simulink model "r2_deng_tvg"  (R2012b)
(part 3 of 46)

      mask prompts: io_dir "I/O direction"; io_delay "I/O delay"; sample_period "Sample period"; names "Name:"; bitwidths "Bitwidth:"; arith_types "Type (ufix=0, fix=1, bool=2):"; bin_pts "Binary pt:"; show_format "Print format string?"
      mask init:
      | swreg_init(gcb)
      settings: AttributesFormatString=1input:uf32.0,
      mask TypeOptions mode: one value | fields of equal size | fields of arbitrary size
      mask Callback mode: swreg_cb(gcb);
      mask TypeOptions io_dir: To Processor | From Processor
      mask Callback io_dir:
      | mask_enables = get_param(gcb, 'MaskEnables');
      | mask_names = get_param(gcb, 'MaskNames');
      | if strcmp(get_param(gcb, 'io_dir'), 'To Processor'),
      |     mask_enables{ismember(mask_names, 'sample_period')} = 'off';
      | else
      |     mask_enables{ismember(mask_names, 'sample_period')} = 'on';
      | end
      | set_param(gcb, 'MaskEnables', mask_enables);
      mask Callback bitwidths:
      | blk = gcb;
      | mode = get_param(blk, 'mode');
      | current_widths = eval(get_param(blk, 'bitwidths'));
      | if (strcmp(mode, 'one value') || strcmp(mode, 'fields of equal size')) && (length(current_widths) > 1),
      |     error('Only one width may be specified for this mode.');
      | elseif strcmp(mode, 'fields of arbitrary size')
      |     current_names = textscan(strtrim(strrep(strrep(get_param(blk, 'names'), ']', ''), '[', '')), '%s');
      |     current_names = current_names{1};
      |     numios = length(current_names);
      |     if length(current_widths) ~= numios,
      |         error('%d field names specified, but %d widths?', numios, length(current_widths));
      |     end
      | end
      | total_width = 0;
      | for ctr = 1 : length(current_widths),
      |     total_width = total_width + current_widths(ctr);
      | end
      | if total_width > 32,
      |     error('Total width must be 32 or less, set to %d.', total_width);
      | end
      mask Callback arith_types:
      | blk = gcb;
      | mode = get_param(blk, 'mode');
      | current_types = eval(get_param(blk, 'arith_types'));
      | numios = length(current_types);
      | if (strcmp(mode, 'one value') || strcmp(mode, 'fields of equal size')) && (length(current_types) > 1),
      |     error('Only one type may be specified for this mode.');
      | elseif strcmp(mode, 'fields of arbitrary size')
      |     current_names = textscan(strtrim(strrep(strrep(get_param(blk, 'names'), ']', ''), '[', '')), '%s');
      |     current_names = current_names{1};
      |     numios = length(current_names);
      |     if length(current_types) ~= numios,
      |         error('%d field names specified, but %d types?', numios, length(current_types));
      |     end
      | end
      | problem = 0;
      | for ctr = 1 : numios,
      |     t = current_types(ctr);
      |     if (t < 0) || (t > 2),
      |         problem = t;
      |         ctr = numios + 1;
      |     end
      | end
      | if problem ~= 0,
      |     error('Type cannot be %i, must be 0, 1 or 2.', problem);
      | end
      mask Callback bin_pts:
      | blk = gcb;
      | mode = get_param(blk, 'mode');
      | current_bins = eval(get_param(blk, 'bin_pts'));
      | if (strcmp(mode, 'one value') || strcmp(mode, 'fields of equal size')) && (length(current_bins) > 1),
      |     error('Only one binary pt may be specified for this mode.');
      | elseif strcmp(mode, 'fields of arbitrary size')
      |     current_names = textscan(strtrim(strrep(strrep(get_param(blk, 'names'), ']', ''), '[', '')), '%s');
      |     current_names = current_names{1};
      |     numios = length(current_names);
      |     if length(current_bins) ~= numios,
      |         error('%d field names specified, but %d binary pts?', numios, length(current_bins));
      |     end
      | end
  tick_offset_msw : Subsystem  Tag=xps:sw_reg  AncestorBlock=xps_library/software register  mask(swreg){mode=one value, io_dir=From Processor, io_delay=1, sample_period=1, names=reg, bitwidths=32, arith_types=0, bin_pts=0, show_format=on}
      mask prompts: io_dir "I/O direction"; io_delay "I/O delay"; sample_period "Sample period"; names "Name:"; bitwidths "Bitwidth:"; arith_types "Type (ufix=0, fix=1, bool=2):"; bin_pts "Binary pt:"; show_format "Print format string?"
      mask init:
      | swreg_init(gcb)
      settings: AttributesFormatString=1input:uf32.0,
      mask TypeOptions mode: one value | fields of equal size | fields of arbitrary size
      mask Callback mode: swreg_cb(gcb);
      mask TypeOptions io_dir: To Processor | From Processor
      mask Callback io_dir:
      | mask_enables = get_param(gcb, 'MaskEnables');
      | mask_names = get_param(gcb, 'MaskNames');
      | if strcmp(get_param(gcb, 'io_dir'), 'To Processor'),
      |     mask_enables{ismember(mask_names, 'sample_period')} = 'off';
      | else
      |     mask_enables{ismember(mask_names, 'sample_period')} = 'on';
      | end
      | set_param(gcb, 'MaskEnables', mask_enables);
      mask Callback bitwidths:
      | blk = gcb;
      | mode = get_param(blk, 'mode');
      | current_widths = eval(get_param(blk, 'bitwidths'));
      | if (strcmp(mode, 'one value') || strcmp(mode, 'fields of equal size')) && (length(current_widths) > 1),
      |     error('Only one width may be specified for this mode.');
      | elseif strcmp(mode, 'fields of arbitrary size')
      |     current_names = textscan(strtrim(strrep(strrep(get_param(blk, 'names'), ']', ''), '[', '')), '%s');
      |     current_names = current_names{1};
      |     numios = length(current_names);
      |     if length(current_widths) ~= numios,
      |         error('%d field names specified, but %d widths?', numios, length(current_widths));
      |     end
      | end
      | total_width = 0;
      | for ctr = 1 : length(current_widths),
      |     total_width = total_width + current_widths(ctr);
      | end
      | if total_width > 32,
      |     error('Total width must be 32 or less, set to %d.', total_width);
      | end
      mask Callback arith_types:
      | blk = gcb;
      | mode = get_param(blk, 'mode');
      | current_types = eval(get_param(blk, 'arith_types'));
      | numios = length(current_types);
      | if (strcmp(mode, 'one value') || strcmp(mode, 'fields of equal size')) && (length(current_types) > 1),
      |     error('Only one type may be specified for this mode.');
      | elseif strcmp(mode, 'fields of arbitrary size')
      |     current_names = textscan(strtrim(strrep(strrep(get_param(blk, 'names'), ']', ''), '[', '')), '%s');
      |     current_names = current_names{1};
      |     numios = length(current_names);
      |     if length(current_types) ~= numios,
      |         error('%d field names specified, but %d types?', numios, length(current_types));
      |     end
      | end
      | problem = 0;
      | for ctr = 1 : numios,
      |     t = current_types(ctr);
      |     if (t < 0) || (t > 2),
      |         problem = t;
      |         ctr = numios + 1;
      |     end
      | end
      | if problem ~= 0,
      |     error('Type cannot be %i, must be 0, 1 or 2.', problem);
      | end
      mask Callback bin_pts:
      | blk = gcb;
      | mode = get_param(blk, 'mode');
      | current_bins = eval(get_param(blk, 'bin_pts'));
      | if (strcmp(mode, 'one value') || strcmp(mode, 'fields of equal size')) && (length(current_bins) > 1),
      |     error('Only one binary pt may be specified for this mode.');
      | elseif strcmp(mode, 'fields of arbitrary size')
      |     current_names = textscan(strtrim(strrep(strrep(get_param(blk, 'names'), ']', ''), '[', '')), '%s');
      |     current_names = current_names{1};
      |     numios = length(current_names);
      |     if length(current_bins) ~= numios,
      |         error('%d field names specified, but %d binary pts?', numios, length(current_bins));
      |     end
      | end
  ticks_since_mrst : Subsystem
  tvg_spead_time_with_pkt_ctr : Subsystem  mask{packetlen_bits=9}
      mask prompts: packetlen_bits "Packet length, num 80-bit words (2^?):"
  wng0 : Subsystem
  wng1 : Subsystem
  wng_corr : Subsystem
  xsg : xps_library/XSG core config  Tag=xps:xsg  hw_sys=ROACH2:sx475t  clk_src=sys_clk  ROACH_clk_src=sys_clk  ROACH2_clk_src=sys_clk  MKDIG_clk_src=sys_clk  clk_rate=1712/8  sample_period=1  synthesis_tool=XST
  tag scope: local_time=global, spead_data0=global, spead_data1=global, spead_data2=global, spead_data3=global, spead_eof0=global, spead_eof1=global, spead_eof2=global, spead_eof3=global, spead_valid0=global, spead_valid1=global, spead_valid2=global, spead_valid3=global, up_cnt_rst=global
  wires:
  [tvg_select0] -> Delay102/1
  Mux/1 -> Assert/1  "d80_0"
  fifo0/1(fifo_data80) -> pipeline96/1(d)  "data00"
  fifo0/2(fifo_dv) -> Gateway Out/1, pipeline97/1(d)  "dv00"
  fifo0/3(word_start) -> Gateway Out2/1, pipeline98/1(d)  "ws00"
  fifo0/4(pkt_start) -> Gateway Out4/1, pipeline99/1(d)  "ps00"
  gbe_porttx/1(in_reg) -> pipeline16/1(d), pipeline15/1(d)
  Constant9/1 -> gbe_porttx/1(sim_1)
  Constant10/1 -> gbe_iptx0/1(sim_1)
  Constant12/1 -> gbe_iptx1/1(sim_1)
  Constant13/1 -> gbe_iptx2/1(sim_1)
  Constant14/1 -> gbe_iptx3/1(sim_1)
  Constant15/1 -> digitiser_id/1(sim_1)
  Constant17/1 -> receptor_id/1(sim_1)
  fifo0/5(fifo_full) -> Terminator16/1  "full00"
  fifo0/6(fifo_empty) -> Terminator23/1  "empty00"
  fifo1/1(fifo_data80) -> pipeline100/1(d)  "data01"
  fifo1/2(fifo_dv) -> Gateway Out1/1, pipeline101/1(d)  "dv01"
  fifo1/3(word_start) -> Gateway Out3/1, pipeline102/1(d)  "ws01"
  fifo1/4(pkt_start) -> Gateway Out5/1, pipeline103/1(d)  "ps01"
  pack_80_64_01/3(data64) -> pipeline117/1(d)  "d64_00"
  pack_80_64_01/2(valid64) -> pipeline116/1(d)  "v64_01"
  pack_80_64_01/1(ready64) -> pipeline115/1(d)  "r64_01"
  fifo1/5(fifo_full) -> Terminator18/1
  fifo1/6(fifo_empty) -> Terminator20/1
  Inverter/1 -> fifo1/2(fifo_we_en)
  Constant16/1 -> digitiser_id/2(sim_2)
  receptor_id/1(in_receptor_id) -> bus_create/3(in3)
  Constant6/1 -> receptor_id/2(sim_2)
  Constant19/1 -> receptor_id/3(sim_3)
  [hdr_0x3101] -> bus_create9/1(in1)
  [pol0_id] -> bus_create9/2(in2)
  [hdr_0x3101] -> bus_create1/1(in1)
  [pol0_id] -> bus_create1/2(in2)
  [speadtime0] -> spead_pack0/8(hdr5_0x1600_DIR), spead_pack0/4(hdr_heap_id)  "timein0"
  bus_create9/1(bus_out) -> spead_pack0/9(hdr6_0x3101_DIR)
  [status0] -> spead_pack0/10(hdr7_0x3102_DIR)
  bus_create1/1(bus_out) -> spead_pack1/9(hdr6_0x3101_DIR)
  [status1] -> spead_pack1/10(hdr7_0x3102_DIR)
  Mux3/1 -> Delay10/1, Delay11/1, Delay12/1, Delay1/1  "status0"
  [tvg_ltime] -> fifo_select/1(localtime)
  fifo_select/1(select) -> Delay3/1  "fifo_select"
  Delay3/1 -> [fifoselect], Inverter/1, fifo0/2(fifo_we_en)  "fifoselect"
  [speadtime1] -> spead_pack1/4(hdr_heap_id), spead_pack1/8(hdr5_0x1600_DIR)  "timein1"
  pack_80_64_00/1(ready64) -> pipeline112/1(d)  "r64_00"
  pack_80_64_00/2(valid64) -> pipeline113/1(d)  "v64_00"
  pack_80_64_00/3(data64) -> pipeline114/1(d)  "d64_00"
  [spead_heapsize] -> spead_pack0/5(hdr_heap_size)
  [spead_heapoffset] -> spead_pack0/6(hdr_heap_offset)
  [spead_pktlen] -> spead_pack0/7(hdr_pkt_len_words)
  [spead_heapsize] -> spead_pack1/5(hdr_heap_size)
  [spead_heapoffset] -> spead_pack1/6(hdr_heap_offset)
  [spead_pktlen] -> spead_pack1/7(hdr_pkt_len_words)
  [masked_time] -> Delay128/1
  Assert/1 -> fifo1/1(data80), fifo0/1(data80)
  tvg_spead_time_with_pkt_ctr/1(local_time) -> Delay131/1
  tvg_spead_time_with_pkt_ctr/3(tvg_data_pol0) -> Delay133/1
  tvg_spead_time_with_pkt_ctr/4(tvg_data_pol1) -> Delay134/1
  tvg_spead_time_with_pkt_ctr/2(spead_time) -> Delay132/1
  spead_pack1/4(data_overflow) -> Terminator15/1
  [adc_data_offset] -> spead_pack0/11(hdr8_0x3300)
  [adc_data_offset] -> spead_pack1/11(hdr8_0x3300)
  Constant26/1 -> [spead_heapsize]
  Constant27/1 -> [spead_pktlen]
  Constant45/1 -> [spead_heapoffset]
  spead_pack0/4(data_overflow) -> Terminator12/1
  spead_pack0/3(eof) -> pipeline56/1(d)
  spead_pack0/1(data_out) -> pipeline54/1(d)  "packd"
  spead_pack0/2(valid_out) -> pipeline55/1(d)  "packv"
  spead_pack1/1(data_out) -> pipeline57/1(d)
  spead_pack1/2(valid_out) -> pipeline58/1(d)
  spead_pack1/3(eof) -> pipeline59/1(d)
  Delay4/1 -> Register6/1, Register5/1  "tvgtime"
  [fifoselect] -> Inverter2/1, edge_detect5/1(in)
  Register5/1 -> [speadtime0]  "speadtime0"
  Inverter2/1 -> edge_detect6/1(in)
  edge_detect5/1(out) -> Register5/2
  edge_detect6/1(out) -> Register6/2
  Register6/1 -> [speadtime1]  "speadtime1"
  [tvg_stime] -> Delay4/1
  Constant8/1 -> [adc_data_offset]
  [mrst] -> ticks_since_mrst/1(reset)
  [sync] -> ticks_since_mrst/2(sync)
  ticks_since_mrst/1(time64) -> [local_time]  "localtime"
  [msync] -> [sync]  "sync"
  edge_detect2/1(out) -> [mrst]  "mrst"
  edge_detect1/1(out) -> [msync]  "msync"
  edge_detect4/1(out) -> [clr_status]  "clr_status"
  [local_time] -> slice1/1, slice2/1
  edge_detect3/1(out) -> [up_cnt_rst]  "mrst"
  Constant28/1 -> control/3(sim_3)
  Constant44/1 -> control/1(sim_1)
  Constant24/1 -> control/2(sim_2)
  Constant33/1 -> control/6(sim_6)
  Constant30/1 -> control/5(sim_5)
  Constant36/1 -> control/4(sim_4)
  Pulse Generator/1 -> control/8(sim_8)
  [tick_offset] -> ticks_since_mrst/3(offset)
  edge_detect10/1(out) -> [load_tick_offset]  "mrst"
  Constant20/1 -> control/9(sim_9)
  digitiser_id/1(in_digitiser_serial) -> bus_create/1(in1)
  digitiser_id/2(in_digitiser_type) -> bus_create/2(in2)
  Constant43/1 -> flag_setup/3(sim_3)
  Constant42/1 -> flag_setup/2(sim_2)
  Constant39/1 -> flag_setup/1(sim_1)
  Counter Free-Running3/1 -> Relational Operator4/2
  Constant48/1 -> Relational Operator4/1
  Relational Operator4/1 -> flag_setup/4(sim_4)
  Constant52/1 -> start_flag_msw/1(sim_1)
  Constant53/1 -> start_flag_lsw/1(sim_1)
  Constant51/1 -> end_flag_msw/1(sim_1)
  Constant50/1 -> end_flag_lsw/1(sim_1)
  Concat4/1 -> Delay49/1  "starttime"
  Concat5/1 -> Delay50/1  "stoptime"
  [flag_start_time] -> Delay46/1
  [local_time] -> Delay45/1, Delay47/1
  [flag_end_time] -> Delay48/1, Delay51/1
  Relational/1 -> Logical2/2  "start_okay"
  [flag_armed] -> Delay44/1
  Relational1/1 -> Logical4/2  "end_okay"
  Logical2/1 -> Delay23/1  "start_okay"
  Logical4/1 -> Logical3/1  "end_okay"
  edge_detect9/1(out) -> [load_flag_time]  "loadtimes"
  Constant4/1 -> Register1/1
  edge_detect8/1(out) -> [reset_flag_time]  "rst"
  [reset_flag_time] -> Register1/2
  [load_flag_time] -> Register1/3
  Register1/1 -> [flag_armed]  "armed"
  Relational Operator3/1 -> flag_setup/5(sim_5)
  Relational2/1 -> Delay22/1  "zero_stop"
  Constant2/1 -> Relational2/2
  Logical3/1 -> Logical1/2  "eokay"
  Counter Free-Running2/1 -> Relational Operator3/2
  Constant5/1 -> Relational Operator3/1
  Logical5/1 -> sample_masking/2(den_in)
  Constant49/1 -> start_time_msw/1(sim_1)
  Constant54/1 -> start_time_lsw/1(sim_1)
  Constant3/1 -> end_time_msw/1(sim_1)
  Constant11/1 -> end_time_lsw/1(sim_1)
  Relational3/1 -> Logical6/2  "start_okay"
  Relational4/1 -> Logical8/2  "end_okay"
  [start_time] -> Delay39/1
  Relational6/1 -> Delay15/1  "first_sample"
  [end_time] -> Delay41/1
  Relational7/1 -> Delay16/1  "last_sample"
  [sample_end] -> sample_masking/6(sample_end)
  [sample_start] -> sample_masking/5(sample_start)
  sample_masking/2(den_out) -> Delay126/1  "enable"
  sample_masking/3(data_mask) -> Delay127/1  "mask"
  edge_detect11/1(out) -> [reset_en_time]  "reset_en_time"
  Relational Operator5/1 -> control_output/2(sim_2)
  Counter Free-Running4/1 -> Relational Operator6/2, Relational Operator5/2
  Constant38/1 -> Relational Operator5/1
  edge_detect12/1(out) -> [load_en_time]  "load_en_time"
  Concat/1 -> Delay42/1
  Concat1/1 -> Delay43/1
  Constant22/1 -> Register2/1
  [reset_en_time] -> Register2/2
  [load_en_time] -> Register2/3
  Register2/1 -> [en_armed]  "armed"
  Logical6/1 -> Delay17/1  "start_okay"
  Logical8/1 -> Logical7/1  "end_okay"
  Logical7/1 -> Logical5/2
  Constant34/1 -> Delay37/1
  Relational5/1 -> Delay14/1
  Constant29/1 -> control_output/3(sim_3)
  Constant47/1 -> control_output/4(sim_4)
  Constant31/1 -> Relational Operator6/1
  Relational Operator6/1 -> control_output/1(sim_1)
  [data_enable] -> Delay129/1
  [sample_mask] -> Delay130/1
  Constant23/1 -> Mux3/2
  [adc_count] -> Concat3/1
  [adc_flag] -> Concat3/3
  [ndiode_flag] -> Concat3/4
  Constant55/1 -> Concat3/2
  Concat3/1 -> Mux3/3
  [flag_en] -> Mux3/1
  Constant46/1 -> tick_offset_msw/1(sim_1)
  Constant7/1 -> tick_offset_lsw/1(sim_1)
  Concat2/1 -> Register3/1
  [load_tick_offset] -> Register3/2
  Register3/1 -> [tick_offset]
  Delay1/1 -> [status0]
  fifo2/1(fifo_data80) -> pipeline104/1(d)  "data00"
  fifo2/2(fifo_dv) -> pipeline105/1(d)  "dv00"
  fifo2/3(word_start) -> pipeline106/1(d)  "ws00"
  fifo2/4(pkt_start) -> pipeline107/1(d)  "ps00"
  fifo2/5(fifo_full) -> Terminator3/1  "full00"
  fifo2/6(fifo_empty) -> Terminator6/1  "empty00"
  fifo3/1(fifo_data80) -> pipeline108/1(d)  "data01"
  fifo3/2(fifo_dv) -> pipeline109/1(d)  "dv01"
  fifo3/3(word_start) -> pipeline110/1(d)  "ws01"
  fifo3/4(pkt_start) -> pipeline111/1(d)  "ps01"
  pack_80_64_2/3(data64) -> pipeline123/1(d)  "d64_00"
  pack_80_64_2/2(valid64) -> pipeline122/1(d)  "v64_01"
  pack_80_64_2/1(ready64) -> pipeline121/1(d)  "r64_01"
  fifo3/5(fifo_full) -> Terminator4/1
  fifo3/6(fifo_empty) -> Terminator5/1
  [hdr_0x3101] -> bus_create3/1(in1)
  [pol1_id] -> bus_create3/2(in2)
  [hdr_0x3101] -> bus_create2/1(in1)
  [pol1_id] -> bus_create2/2(in2)
  [speadtime0] -> spead_pack2/4(hdr_heap_id), spead_pack2/8(hdr5_0x1600_DIR)  "timein0"
  bus_create3/1(bus_out) -> spead_pack2/9(hdr6_0x3101_DIR)
  [status2] -> spead_pack2/10(hdr7_0x3102_DIR)
  bus_create2/1(bus_out) -> spead_pack3/9(hdr6_0x3101_DIR)
  [status3] -> spead_pack3/10(hdr7_0x3102_DIR)
  [speadtime1] -> spead_pack3/8(hdr5_0x1600_DIR), spead_pack3/4(hdr_heap_id)  "timein1"
  pack_80_64_1/1(ready64) -> pipeline118/1(d)  "r64_00"
  pack_80_64_1/2(valid64) -> pipeline119/1(d)  "v64_00"
  pack_80_64_1/3(data64) -> pipeline120/1(d)  "d64_00"
  [spead_heapsize] -> spead_pack2/5(hdr_heap_size)
  [spead_heapoffset] -> spead_pack2/6(hdr_heap_offset)
  [spead_pktlen] -> spead_pack2/7(hdr_pkt_len_words)
  [spead_heapsize] -> spead_pack3/5(hdr_heap_size)
  [spead_heapoffset] -> spead_pack3/6(hdr_heap_offset)
  [spead_pktlen] -> spead_pack3/7(hdr_pkt_len_words)
  spead_pack3/4(data_overflow) -> Terminator2/1
  [adc_data_offset] -> spead_pack2/11(hdr8_0x3300)
  [adc_data_offset] -> spead_pack3/11(hdr8_0x3300)
  spead_pack2/4(data_overflow) -> Terminator1/1
  spead_pack2/3(eof) -> pipeline62/1(d)
  spead_pack2/1(data_out) -> pipeline60/1(d)  "packd"
  spead_pack2/2(valid_out) -> pipeline61/1(d)  "packv"
  spead_pack3/1(data_out) -> pipeline63/1(d)
  spead_pack3/2(valid_out) -> pipeline64/1(d)
  spead_pack3/3(eof) -> pipeline65/1(d)
  Inverter1/1 -> fifo3/2(fifo_we_en)
  [tvg_select1] -> Delay106/1
  Mux1/1 -> Assert1/1  "d80_0"
  [data_80_1] -> Delay109/1
  [tvg_pol1] -> Delay108/1
  Assert1/1 -> fifo3/1(data80), fifo2/1(data80)
  [fifoselect] -> Inverter1/1, fifo2/2(fifo_we_en)
  [gbe0_txen] -> Logical13/1, Logical10/2
  Logical10/1 -> pipeline86/1(d)
  [gbe_port0] -> gbe0/5(tx_dest_port)
  Constant56/1 -> gbe0/8(rx_overrun_ack), gbe0/7(rx_ack)
  [spead_valid0] -> Logical10/1
  pipeline83/1(q) -> gbe0/2(tx_data)
  [gbe_ip0] -> gbe0/4(tx_dest_ip)
  [gbe_rst] -> pipeline68/1(d)
  [gbe1_txen] -> Logical14/1, Logical9/2
  Logical9/1 -> pipeline85/1(d)
  [gbe_port1] -> gbe1/5(tx_dest_port)
  Constant18/1 -> gbe1/8(rx_overrun_ack), gbe1/7(rx_ack)
  [spead_valid1] -> Logical9/1
  pipeline80/1(q) -> gbe1/2(tx_data)
  [gbe_ip1] -> gbe1/4(tx_dest_ip)
  [gbe_rst] -> pipeline70/1(d)
  [gbe2_txen] -> Logical15/1, Logical12/2
  Logical12/1 -> pipeline82/1(d)
  [gbe_port2] -> gbe2/5(tx_dest_port)
  Constant25/1 -> gbe2/8(rx_overrun_ack), gbe2/7(rx_ack)
  [spead_valid2] -> Logical12/1
  pipeline77/1(q) -> gbe2/2(tx_data)
  [gbe_ip2] -> gbe2/4(tx_dest_ip)
  [gbe3_txen] -> Logical16/1, Logical11/2
  Logical11/1 -> pipeline75/1(d)
  [gbe_port3] -> gbe3/5(tx_dest_port)
  Constant21/1 -> gbe3/8(rx_overrun_ack), gbe3/7(rx_ack)
  [spead_data3] -> pipeline74/1(d)
  [gbe_ip3] -> gbe3/4(tx_dest_ip)
  [clr_status] -> pipeline69/1(d)
  [clr_status] -> pipeline71/1(d)
  [spead_eof0] -> Logical13/2
  [spead_eof1] -> Logical14/2
  Logical15/1 -> pipeline87/1(d)
  [spead_eof2] -> Logical15/2
  Logical16/1 -> pipeline76/1(d)
  [spead_eof3] -> Logical16/2
  gbe0/1(led_up) -> Terminator77/1
  gbe0/2(led_rx) -> Terminator67/1
  gbe0/3(led_tx) -> Terminator72/1
  gbe0/4(tx_afull) -> Terminator73/1
  gbe0/5(tx_overflow) -> Terminator75/1
  gbe0/6(rx_data) -> Terminator66/1
  gbe0/7(rx_valid) -> Terminator68/1
  gbe0/8(rx_source_ip) -> Terminator69/1
  gbe0/9(rx_source_port) -> Terminator70/1
  gbe0/10(rx_end_of_frame) -> Terminator71/1
  gbe0/11(rx_bad_frame) -> Terminator74/1
  gbe0/12(rx_overrun) -> Terminator76/1
  gbe1/1(led_up) -> Terminator13/1
  gbe1/2(led_rx) -> Terminator8/1
  gbe1/3(led_tx) -> Terminator40/1
  gbe1/4(tx_afull) -> Terminator43/1
  gbe1/5(tx_overflow) -> Terminator10/1
  gbe1/6(rx_data) -> Terminator7/1
  gbe1/7(rx_valid) -> Terminator9/1
  gbe1/8(rx_source_ip) -> Terminator34/1
  gbe1/9(rx_source_port) -> Terminator37/1
  gbe1/10(rx_end_of_frame) -> Terminator38/1
  gbe1/11(rx_bad_frame) -> Terminator46/1
  gbe1/12(rx_overrun) -> Terminator11/1
  gbe2/1(led_up) -> Terminator21/1
  gbe2/2(led_rx) -> Terminator22/1
  gbe2/3(led_tx) -> Terminator28/1
  gbe2/4(tx_afull) -> Terminator29/1
  gbe2/5(tx_overflow) -> Terminator17/1
  gbe2/6(rx_data) -> Terminator14/1
  gbe2/7(rx_valid) -> Terminator24/1
  gbe2/8(rx_source_ip) -> Terminator25/1
  gbe2/9(rx_source_port) -> Terminator26/1
  gbe2/10(rx_end_of_frame) -> Terminator27/1
  gbe2/11(rx_bad_frame) -> Terminator30/1
  gbe2/12(rx_overrun) -> Terminator19/1
  gbe3/1(led_up) -> Terminator35/1
  gbe3/2(led_rx) -> Terminator36/1
  gbe3/3(led_tx) -> Terminator45/1
  gbe3/4(tx_afull) -> Terminator47/1
  gbe3/5(tx_overflow) -> Terminator32/1
  gbe3/6(rx_data) -> Terminator31/1
  gbe3/7(rx_valid) -> Terminator39/1
  gbe3/8(rx_source_ip) -> Terminator41/1
  gbe3/9(rx_source_port) -> Terminator42/1
  gbe3/10(rx_end_of_frame) -> Terminator44/1
  gbe3/11(rx_bad_frame) -> Terminator48/1
  gbe3/12(rx_overrun) -> Terminator33/1
  Logical13/1 -> pipeline84/1(d)
  Logical14/1 -> pipeline81/1(d)
  [spead_data0] -> pipeline83/1(d)
  [spead_data1] -> pipeline80/1(d)
  [spead_data2] -> pipeline77/1(d)
  [spead_valid3] -> Logical11/1
  scale_wng1/1(in_scale) -> pipeline43/1(d)
  scale_wng_corr/1(in_scale) -> pipeline42/1(d)
  wng0/1(bus_out) -> Slice/1, pipeline78/1(d)
  wng1/1(bus_out) -> pipeline89/1(d)
  cwg0/1(bus_out) -> Slice1/1, pipeline90/1(d)
  cwg_corr/1(bus_out) -> pipeline92/1(d), pipeline91/1(d)
  cwg1/1(bus_out) -> pipeline93/1(d)
  bus_addsub/1(dout) -> Delay105/1
  bus_addsub2/1(dout) -> Delay6/1
  bus_addsub3/1(dout) -> Delay9/1
  bus_addsub1/1(dout) -> Delay5/1
  bus_addsub4/1(dout) -> bus_convert6/1(din)
  bus_mult/1(a*b) -> Slice4/1, bus_convert/1(din)
  bus_addsub5/1(dout) -> bus_convert7/1(din)
  bus_mult1/1(a*b) -> bus_convert1/1(din)
  scale_out1/1(in_scale) -> pipeline52/1(d)
  Constant35/1 -> scale_wng0/1(sim_1)
  Constant1/1 -> scale_wng_corr/1(sim_1)
  freq_cwg0/2(in_scale) -> pipeline44/1(d)
  Constant64/1 -> freq_cwg0/1(sim_1)
  Constant57/1 -> scale_out0/1(sim_1)
  Constant58/1 -> scale_out1/1(sim_1)
  freq_cwg1/2(in_scale) -> pipeline48/1(d)
  freq_cwg1/1(in_frequency) -> pipeline49/1(d)
  freq_cwg_corr/2(in_scale) -> pipeline46/1(d)
  pipeline21/1(q) -> edge_detect12/1(in)
  pipeline22/1(q) -> edge_detect11/1(in)
  pipeline23/1(q) -> [sample_start]
  pipeline24/1(q) -> [sample_end]
  Delay42/1 -> [start_time]
  Delay43/1 -> [end_time]
  Delay49/1 -> [flag_start_time]
  Delay50/1 -> [flag_end_time]
  pipeline41/1(q) -> wng0/1(scale_16_14)
  pipeline42/1(q) -> wng_corr/1(scale_16_14)
  pipeline43/1(q) -> wng1/1(scale_16_14)
  pipeline10/1(q) -> [gbe_ip3]
  pipeline11/1(q) -> [gbe_ip2]
  pipeline13/1(q) -> [gbe_ip0]
  pipeline9/1(q) -> [gbe_port0]
  Delay102/1 -> Mux/1
  Delay103/1 -> Mux/2
  Delay104/1 -> Mux/3
  Delay106/1 -> Mux1/1
  Delay126/1 -> [data_enable]
  Delay127/1 -> [sample_mask]
  Delay128/1 -> tvg_spead_time_with_pkt_ctr/1(localtime64)
  Delay129/1 -> tvg_spead_time_with_pkt_ctr/2(data_enable)
  Delay130/1 -> tvg_spead_time_with_pkt_ctr/3(data_mask)
  Delay131/1 -> [tvg_ltime]
  Delay132/1 -> [tvg_stime]
  Delay133/1 -> [tvg_pol0]
  Delay134/1 -> [tvg_pol1]
  [tvg_pol0] -> Delay103/1
  [data_80_0] -> Delay104/1
  Delay109/1 -> Mux1/3
  Delay108/1 -> Mux1/2
  Delay105/1 -> bus_convert2/1(din)
  Delay5/1 -> bus_convert3/1(din)
  Delay6/1 -> bus_convert4/1(din)
  Delay9/1 -> bus_convert5/1(din)
  Delay139/1 -> bus_addsub4/1(a)
  Delay7/1 -> bus_addsub5/1(a)
  Delay8/1 -> bus_addsub5/2(b)
  pipeline25/1(q) -> Concat/1
  pipeline26/1(q) -> Concat/2
  pipeline27/1(q) -> Concat1/1
  pipeline28/1(q) -> Concat1/2
  pipeline29/1(q) -> [hdr_0x3101]
  pipeline30/1(q) -> [pol0_id]
  pipeline31/1(q) -> [pol1_id]
  control/1(in_up_cnt_rst) -> pipeline/1(d)
  pipeline/1(q) -> edge_detect3/1(in)
  control/2(in_tvg_select0) -> pipeline1/1(d)
  control/3(in_tvg_select1) -> pipeline2/1(d)
  control/4(in_clr_status) -> pipeline3/1(d)
  control/5(in_gbe_rst) -> pipeline4/1(d)
  control/6(in_gbe_txen) -> pipeline5/1(d)
  control/7(in_msync) -> pipeline6/1(d)
  control/8(in_mrst) -> pipeline7/1(d)
  control/9(in_load_tick_offset) -> pipeline8/1(d)
  pipeline8/1(q) -> edge_detect10/1(in)
  pipeline7/1(q) -> edge_detect2/1(in)
  pipeline6/1(q) -> edge_detect1/1(in)
  pipeline4/1(q) -> [gbe_rst]
  pipeline3/1(q) -> edge_detect4/1(in)
  pipeline2/1(q) -> [tvg_select1]
  pipeline1/1(q) -> [tvg_select0]
  pipeline12/1(q) -> [gbe_ip1]
  pipeline16/1(q) -> pipeline124/1(d), pipeline125/1(d)
  pipeline14/1(q) -> [gbe_port1]
  gbe_iptx0/1(in_reg) -> pipeline13/1(d)
  gbe_iptx1/1(in_reg) -> pipeline12/1(d)
  gbe_iptx2/1(in_reg) -> pipeline11/1(d)
  gbe_iptx3/1(in_reg) -> pipeline10/1(d)
  tick_offset_msw/1(in_reg) -> pipeline17/1(d)
  pipeline17/1(q) -> Concat2/1
  tick_offset_lsw/1(in_reg) -> pipeline18/1(d)
  pipeline18/1(q) -> Concat2/2
  slice1/1 -> pipeline20/1(d)
  pipeline20/1(q) -> local_time_lsw/1(out_reg)
  slice2/1 -> pipeline19/1(d)
  pipeline19/1(q) -> local_time_msw/1(out_reg)
  end_time_lsw/1(in_reg) -> pipeline28/1(d)
  end_time_msw/1(in_reg) -> pipeline27/1(d)
  start_time_lsw/1(in_reg) -> pipeline26/1(d)
  start_time_msw/1(in_reg) -> pipeline25/1(d)
  control_output/4(in_sample_end) -> pipeline24/1(d)
  control_output/3(in_sample_start) -> pipeline23/1(d)
  control_output/2(in_reset_en_time) -> pipeline22/1(d)
  control_output/1(in_load_en_time) -> pipeline21/1(d)
  bus_create/1(bus_out) -> pipeline29/1(d)
  receptor_id/2(in_pol0_id) -> pipeline30/1(d)
  receptor_id/3(in_pol1_id) -> pipeline31/1(d)
  flag_setup/1(in_adc_count) -> pipeline32/1(d)
  flag_setup/2(in_adc_flag) -> pipeline33/1(d)
  flag_setup/3(in_ndiode_flag) -> pipeline34/1(d)
  flag_setup/4(in_load_flags) -> pipeline35/1(d)
  flag_setup/5(in_reset_flags) -> pipeline36/1(d)
  pipeline36/1(q) -> edge_detect8/1(in)
  pipeline35/1(q) -> edge_detect9/1(in)
  pipeline34/1(q) -> [ndiode_flag]
  pipeline33/1(q) -> [adc_flag]
  pipeline32/1(q) -> [adc_count]
  start_flag_msw/1(in_reg) -> pipeline37/1(d)
  pipeline37/1(q) -> Concat4/1
  start_flag_lsw/1(in_reg) -> pipeline38/1(d)
  pipeline38/1(q) -> Concat4/2
  end_flag_msw/1(in_reg) -> pipeline39/1(d)
  pipeline39/1(q) -> Concat5/1
  end_flag_lsw/1(in_reg) -> pipeline40/1(d)
  pipeline40/1(q) -> Concat5/2
  freq_cwg_corr/1(in_frequency) -> pipeline47/1(d)
  pipeline53/1(q) -> bus_mult1/1(a)
  pipeline52/1(q) -> bus_mult1/2(b)
  pipeline51/1(q) -> bus_mult/2(b)
  pipeline50/1(q) -> bus_mult/1(a)
  pipeline54/1(q) -> slice4/1, [spead_data0]
  pipeline55/1(q) -> [spead_valid0]
  pipeline56/1(q) -> [spead_eof0]
  pipeline57/1(q) -> [spead_data1]
  pipeline58/1(q) -> [spead_valid1]
  pipeline59/1(q) -> [spead_eof1]
  pipeline60/1(q) -> [spead_data2]
  pipeline61/1(q) -> [spead_valid2]
  pipeline62/1(q) -> [spead_eof2]
  pipeline63/1(q) -> [spead_data3]
  pipeline64/1(q) -> [spead_valid3]
  pipeline65/1(q) -> [spead_eof3]
  [gbe_rst] -> pipeline66/1(d)
  pipeline66/1(q) -> gbe0/1(rst)
  [clr_status] -> pipeline67/1(d)
  pipeline67/1(q) -> gbe0/9(debug_rst)
  pipeline68/1(q) -> gbe1/1(rst)
  pipeline69/1(q) -> gbe1/9(debug_rst)
  pipeline70/1(q) -> gbe2/1(rst)
  pipeline71/1(q) -> gbe2/9(debug_rst)
  [gbe_rst] -> pipeline72/1(d)
  pipeline72/1(q) -> gbe3/1(rst)
  [clr_status] -> pipeline73/1(d)
  pipeline73/1(q) -> gbe3/9(debug_rst)
  pipeline86/1(q) -> gbe0/3(tx_valid)
  pipeline84/1(q) -> gbe0/6(tx_end_of_frame)
  pipeline85/1(q) -> gbe1/3(tx_valid)
  pipeline81/1(q) -> gbe1/6(tx_end_of_frame)
  pipeline82/1(q) -> gbe2/3(tx_valid)
  pipeline87/1(q) -> gbe2/6(tx_end_of_frame)
  pipeline74/1(q) -> gbe3/2(tx_data)
  pipeline75/1(q) -> gbe3/3(tx_valid)
  pipeline76/1(q) -> gbe3/6(tx_end_of_frame)
  pipeline78/1(q) -> bus_addsub/1(a)
  pipeline79/1(q) -> bus_addsub/2(b)
  pipeline88/1(q) -> bus_addsub1/1(a)
  wng_corr/1(bus_out) -> pipeline79/1(d), pipeline88/1(d)
  pipeline89/1(q) -> bus_addsub1/2(b)
  pipeline90/1(q) -> bus_addsub2/1(a)
  pipeline91/1(q) -> bus_addsub2/2(b)
  pipeline92/1(q) -> bus_addsub3/1(a)
  pipeline93/1(q) -> bus_addsub3/2(b)
  pipeline94/1(q) -> [data_80_0]
  pipeline95/1(q) -> [data_80_1]
  pipeline96/1(q) -> pack_80_64_00/1(data80)
  pipeline97/1(q) -> pack_80_64_00/2(valid80)
  pipeline98/1(q) -> pack_80_64_00/3(word_start)
  pipeline99/1(q) -> pack_80_64_00/4(pkt_start)
  pipeline100/1(q) -> pack_80_64_01/1(data80)
  pipeline101/1(q) -> pack_80_64_01/2(valid80)
  pipeline102/1(q) -> pack_80_64_01/3(word_start)
  pipeline103/1(q) -> pack_80_64_01/4(pkt_start)
  pipeline105/1(q) -> pack_80_64_1/2(valid80)
  pipeline104/1(q) -> pack_80_64_1/1(data80)
  pipeline106/1(q) -> pack_80_64_1/3(word_start)
  pipeline107/1(q) -> pack_80_64_1/4(pkt_start)
  pipeline108/1(q) -> pack_80_64_2/1(data80)
  pipeline109/1(q) -> pack_80_64_2/2(valid80)
  pipeline110/1(q) -> pack_80_64_2/3(word_start)
  pipeline111/1(q) -> pack_80_64_2/4(pkt_start)
  pipeline112/1(q) -> spead_pack0/1(data64_ready)
  pipeline113/1(q) -> spead_pack0/2(data64_valid)
  pipeline114/1(q) -> spead_pack0/3(data64)
  pipeline115/1(q) -> spead_pack1/1(data64_ready)
  pipeline116/1(q) -> spead_pack1/2(data64_valid)
  pipeline117/1(q) -> spead_pack1/3(data64)
  pipeline118/1(q) -> spead_pack2/1(data64_ready)
  pipeline119/1(q) -> spead_pack2/2(data64_valid)
  pipeline120/1(q) -> spead_pack2/3(data64)
  pipeline121/1(q) -> spead_pack3/1(data64_ready)
  pipeline122/1(q) -> spead_pack3/2(data64_valid)
  pipeline123/1(q) -> spead_pack3/3(data64)
  pipeline125/1(q) -> [gbe_port2]
  pipeline124/1(q) -> [gbe_port3]
  pipeline15/1(q) -> pipeline14/1(d), pipeline9/1(d)
  Delay2/1 -> bus_addsub4/2(b)
  Delay12/1 -> [status3]
  Delay11/1 -> [status2]
  Delay10/1 -> [status1]
  Delay13/1 -> Logical8/1, Logical6/1
  Delay14/1 -> Logical7/2
  Delay15/1 -> Delay18/1
  Delay16/1 -> Delay19/1
  Delay17/1 -> Logical5/1
  Delay18/1 -> Delay20/1
  Delay19/1 -> Delay21/1
  Delay20/1 -> sample_masking/3(first_samples)
  Delay21/1 -> sample_masking/4(last_samples)
  Delay22/1 -> Logical3/2
  Delay23/1 -> Logical1/1
  Delay24/1 -> Delay25/1
  Delay25/1 -> Delay26/1
  Delay26/1 -> Delay27/1
  Delay27/1 -> sample_masking/1(timei)
  sample_masking/4(flag_valid) -> Delay28/1
  Delay28/1 -> [flag_en]
  Logical1/1 -> sample_masking/7(flag_en)  "flag_en"
  sample_masking/1(timeo) -> Delay29/1
  Delay29/1 -> [masked_time]
  [local_time] -> Delay30/1
  [en_armed] -> Delay31/1
  [local_time] -> Delay32/1, Delay34/1, Delay38/1, Delay40/1
  [start_time] -> Delay33/1
  [end_time] -> Delay35/1, Delay36/1
  Delay30/1 -> Delay24/1
  Delay31/1 -> Delay13/1
  Delay32/1 -> Relational3/1
  Delay33/1 -> Relational3/2
  Delay34/1 -> Relational4/1
  Delay35/1 -> Relational4/2
  Delay36/1 -> Relational5/1
  Delay37/1 -> Relational5/2
  Delay38/1 -> Relational6/1
  Delay39/1 -> Relational6/2
  Delay40/1 -> Relational7/1
  Delay41/1 -> Relational7/2
  Delay44/1 -> Logical4/1, Logical2/1
  Delay45/1 -> Relational/1
  Delay46/1 -> Relational/2
  Delay47/1 -> Relational1/1
  Delay48/1 -> Relational1/2
  Delay51/1 -> Relational2/1
  bus_convert/1(dout) -> Slice5/1, slice5/1, pipeline94/1(d)
  bus_convert1/1(dout) -> pipeline95/1(d)
  Gateway Out/1 -> Scope/1
  Gateway Out1/1 -> Scope/2
  Gateway Out2/1 -> Scope/3
  Gateway Out3/1 -> Scope/4
  Gateway Out4/1 -> Scope/5
  Gateway Out5/1 -> Scope/6
  Pulse Generator1/1 -> control/7(sim_7)
  Slice/1 -> Reinterpret/1
  Slice1/1 -> Reinterpret1/1
  Gateway Out6/1 -> Scope1/1
  Gateway Out7/1 -> Scope1/2
  Reinterpret/1 -> Gateway Out6/1
  Reinterpret1/1 -> Gateway Out7/1
  Slice2/1 -> Reinterpret2/1
  Gateway Out8/1 -> Scope1/3
  Reinterpret2/1 -> Gateway Out8/1
  Slice3/1 -> Reinterpret3/1
  Reinterpret3/1 -> Gateway Out9/1
  Gateway Out9/1 -> Scope1/4
  Slice4/1 -> Reinterpret4/1
  Reinterpret4/1 -> Gateway Out10/1
  Gateway Out10/1 -> Scope1/5
  Slice5/1 -> Reinterpret5/1
  Reinterpret5/1 -> Gateway Out11/1
  Gateway Out11/1 -> Scope1/6
  pipeline45/1(q) -> cwg0/1(freq)
  pipeline44/1(q) -> cwg0/2(scale)
  pipeline47/1(q) -> cwg_corr/1(freq)
  pipeline46/1(q) -> cwg_corr/2(scale)
  pipeline49/1(q) -> cwg1/1(freq)
  pipeline48/1(q) -> cwg1/2(scale)
  bus_convert2/1(dout) -> Slice2/1, Delay139/1
  bus_convert3/1(dout) -> Delay7/1
  bus_convert4/1(dout) -> Delay2/1
  bus_convert5/1(dout) -> Delay8/1
  bus_convert6/1(dout) -> Slice3/1, pipeline50/1(d)
  bus_convert7/1(dout) -> pipeline53/1(d)
  Constant32/1 -> scale_wng1/1(sim_1)
  scale_wng0/1(in_scale) -> pipeline41/1(d)
  Constant59/1 -> scale_wng0/2(sim_2)
  Constant60/1 -> scale_wng_corr/2(sim_2)
  Constant62/1 -> scale_wng1/2(sim_2)
  freq_cwg0/1(in_frequency) -> pipeline45/1(d)
  Constant37/1 -> freq_cwg0/2(sim_2)
  Counter Free-Running1/1 -> freq_cwg1/1(sim_1)
  Constant41/1 -> freq_cwg1/2(sim_2)
  Constant79/1 -> freq_cwg_corr/1(sim_1)
  Constant40/1 -> freq_cwg_corr/2(sim_2)
  scale_out0/1(in_scale) -> pipeline51/1(d)
  Constant61/1 -> scale_out0/2(sim_2)
  Constant63/1 -> scale_out1/2(sim_2)
  Gateway Out12/1 -> To Workspace/1
  Gateway Out13/1 -> To Workspace1/1
  slice4/1 -> Gateway Out12/1
  slice5/1 -> Gateway Out13/1
  pipeline127/1(q) -> Slice6/1
  Slice6/1 -> Convert/1
  Convert/1 -> [pol0_always_on]
  Constant65/1 -> Delay/1
  pipeline131/1(q) -> Slice8/1
  Slice8/1 -> Convert2/1
  Convert2/1 -> [pol0_traffic_trigger]
  [pol0_always_on] -> gbe0_traffic_control/1(always_on)
  [pol0_requested_pkts] -> gbe0_traffic_control/2(requested_pkts)
  [pol0_offset_data] -> gbe0_traffic_control/3(offset_data)
  [mrst] -> gbe0_traffic_control/4(mrst)
  [pol0_traffic_trigger] -> gbe0_traffic_control/5(traffic_trigger)
  gbe0_traffic_control/1(gbe_txen) -> Gateway Out14/1, [gbe0_txen]
  Constant68/1 -> pol1_sample_offset/1(sim_1)
  pipeline129/1(q) -> [pol1_offset_data]
  Constant67/1 -> pol0_sample_offset/1(sim_1)
  pipeline128/1(q) -> [pol0_offset_data]
  Constant69/1 -> pol0_num_pkts/1(sim_1)
  pipeline126/1(q) -> [pol0_requested_pkts]
  Constant73/1 -> pol1_num_pkts/1(sim_1)
  pipeline134/1(q) -> [pol1_requested_pkts]
  pipeline136/1(q) -> Slice7/1
  Slice7/1 -> Convert1/1
  Convert1/1 -> [pol1_always_on]
  [pol0_always_on] -> gbe1_traffic_control/1(always_on)
  [pol0_requested_pkts] -> gbe1_traffic_control/2(requested_pkts)
  [pol0_offset_data] -> gbe1_traffic_control/3(offset_data)
  [mrst] -> gbe1_traffic_control/4(mrst)
  [pol0_traffic_trigger] -> gbe1_traffic_control/5(traffic_trigger)
  [pol1_always_on] -> gbe2_traffic_control/1(always_on)
  [pol1_requested_pkts] -> gbe2_traffic_control/2(requested_pkts)
  [pol1_offset_data] -> gbe2_traffic_control/3(offset_data)
  [mrst] -> gbe2_traffic_control/4(mrst)
  [pol1_traffic_trigger] -> gbe2_traffic_control/5(traffic_trigger)
  gbe2_traffic_control/1(gbe_txen) -> Gateway Out16/1, [gbe2_txen]
  [pol1_always_on] -> gbe3_traffic_control/1(always_on)
  [pol1_requested_pkts] -> gbe3_traffic_control/2(requested_pkts)
  [pol1_offset_data] -> gbe3_traffic_control/3(offset_data)
  [mrst] -> gbe3_traffic_control/4(mrst)
  [pol1_traffic_trigger] -> gbe3_traffic_control/5(traffic_trigger)
  gbe3_traffic_control/1(gbe_txen) -> Gateway Out17/1, [gbe3_txen]
  pipeline5/1(q) -> Terminator49/1
  Constant78/1 -> [gbe_txen]
  gbe1_traffic_control/1(gbe_txen) -> Gateway Out15/1, [gbe1_txen]
  Delay/1 -> pol_traffic_trigger/1(sim_1)
  Gateway Out14/1 -> To Workspace2/1
  Gateway Out15/1 -> To Workspace3/1
  Gateway Out16/1 -> To Workspace4/1
  Gateway Out17/1 -> To Workspace5/1
  Constant66/1 -> pol_tx_always_on/1(sim_1)
  Constant77/1 -> pol_tx_always_on/2(sim_2)
  pol0_num_pkts/1(in_pol0_num_pkts) -> pipeline126/1(d)
  pol1_num_pkts/1(in_pol1_num_pkts) -> pipeline134/1(d)
  pol_tx_always_on/1(in_pol0_tx_always_on) -> pipeline127/1(d)
  pol_tx_always_on/2(in_pol1_tx_always_on) -> pipeline136/1(d)
  pol0_sample_offset/1(in_pol0_sample_offset) -> pipeline128/1(d)
  pol1_sample_offset/1(in_pol1_sample_offset) -> pipeline129/1(d)
  Constant70/1 -> Delay52/1
  Delay52/1 -> pol_traffic_trigger/2(sim_2)
  pol_traffic_trigger/1(in_pol0_tx_trigger) -> pipeline131/1(d)
  pipeline130/1(q) -> Slice9/1
  Slice9/1 -> Convert3/1
  Convert3/1 -> [pol1_traffic_trigger]
  pol_traffic_trigger/2(in_pol1_tx_trigger) -> pipeline130/1(d)
